simulink model "Sim_Uncertain_Delay_iqctest1"  (Simulink 7.3)
settings: Solver=ode45  StartTime=0.0  StopTime=100.0  RelTol=1e-3
settings Model: Creator=MD710  LastModifiedBy=MD710
settings DebuggingCC: SaveWithParameterizedLinksMsg=none  SolverPrmCheckMsg=none  MultiTaskDSMMsg=warning  MultiTaskCondExecSysMsg=none  FcnCallInpInsideContextMsg=Enable All  StrictBusMsg=None
settings HardwareCC: TargetHWDeviceType=32-bit Generic
settings RTWCC: IncludeERTFirstTime=on
settings GRTTargetCC: TargetFcnLib=ansi_tfl_tmw.mat

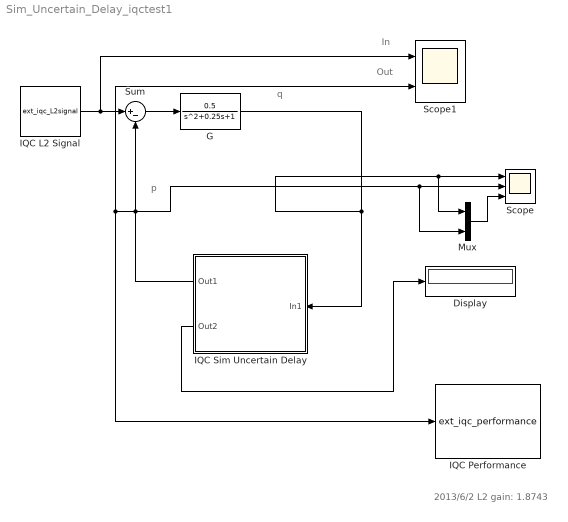
== system Sim_Uncertain_Delay_iqctest1 ==
  note: q
  note: p
  note: 2013/6/2 L2 gain: 1.8743
  note: In
  note: Out
  Display : Display
  G : TransferFcn  Numerator=[0.5]  Denominator=[1 0.25 1]
  IQC L2 Signal : M-S-Function  FunctionName=ext_iqc_L2signal  Parameters=sig_size,sam_time,sig_type,tru_time,sig_amp,sig_fre,user_cus  mask(IQC L2 signal(ver:0.1)){sig_size=1, sam_time=0, sig_type=Step, tru_time=3, sig_amp=1, sig_fre=1, user_cus='2*exp(3*t)'}
      mask prompts: sig_size "Signal Dimension:(Default: 1)"; sam_time "Sample Time:(Default: 0)"; sig_type "Signal Type:"; tru_time "Truncation Time:"; sig_amp "Maximum Amplitude:"; sig_fre "Frequency:"; user_cus "Custom:"
      mask help:
      | Important:
      | In IQC procedure step (as commond iqc_gain_tbx, the task is get
      | L2 gain value), regardless of the user to choose which option (ex sine...),
      | here regarded as generalized L2 signal.
      mask StyleString: edit,edit,popup(Step|Square wave|Sine wave|Custom|Random|External),edit,edit,edit,edit
      mask CallbackString: ||iqc_block_cho(gcb,'L2signal_type')||||
      mask TabNameString: Main,Main,Simulation,Simulation,Simulation,Simulation,Simulation
      mask Display: plot(0:0.1:10,[sin(0:0.1:6.2) zeros(1,38)])
  IQC Performance : M-S-Function  FunctionName=ext_iqc_performance  Parameters=imp_met,save_lin_com,isiqcbode,fre_ran,uselmitool,lmi_par  mask(IQC Performance(ver:0.1)){imp_met=Calculation and Simulation, save_lin_com=off, isiqcbode=off, fre_ran='', uselmitool=lmilab, lmi_par=''}
      mask prompts: imp_met "Implementation Methods"; save_lin_com "Save the Linear File and Command File"; isiqcbode "Display IQC Bode Figure"; fre_ran "Frequency Range:(Default: empty)"; uselmitool "LMI Tool:"; lmi_par "Parameter:(if empty use define)"
      mask help:
      | Important:
      | In IQC toolbox calculate step (as commond iqc_gain_tbx, the task is get
      | L2 gain value), regardless of the user to connect any signal input(Even if
      | not a signal), here regarded as generalized L2 signal.
      |
      | Example 1: setlmioptions('',[0 200 0 0 777])
      | the block parameter is
      | LMI Tool: lmilab
      | Parameter:
      |        [0 200 0 0 777]
      |
      | Example 2: setlmioptions('yalmip','solver','sdpt3','verbose',1)
      | the block parameter is
      | LMI Tool: yalmip
      | Parameter:
      |        {'solver',sdpt3','verbose',1}
      mask Help:
      | <a href="matlab:doc abst_init_iqc;">abst_init_iqc</a>
      | <a href="matlab:doc setlmioptions;">setlmioptions</a>
      | <a href="matlab:doc iqc_gain_tbx;">iqc_gain_tbx</a>
      mask StyleString: popup(Calculation and Simulation|Only Calculation|Only Simulation),checkbox,checkbox,edit,popup(lmilab|yalmip),edit
      mask CallbackString: iqc_block_cho(gcb,'performance_imp')||iqc_block_cho(gcb,'performance_bodefre')|||
      mask TabNameString: Main,Main,Main,Main,LMI,LMI
      mask Display: fprintf('In -> Out \n performance \n L2 gain:\n%4.4f',1.8743);
  IQC Sim Uncertain Delay : Subsystem  mask(IQC Sim Uncertain Delay(ver:0.1)){sou_del=Custom, max_del=0.5, num_ran=1, cus=[0.5], iqc1=on, iqc1_pole=[1 2], iqc1_out='', iqc2=off, iqc2_pole=[], iqc2_out='', iqc3=off, lis_rel='', delay_time=0}
      mask prompts: sou_del "Source of the delay:(Default: Random)"; max_del "Maximum Delay:"; num_ran "The Number of Random:(1 or input_dim)"; cus "Custom:"; iqc1 "iqc_delay(Input,Maximum Delay,Pole)"; iqc1_pole "Pole:(Default: [])"; iqc1_out "Output Variable:(Default: empty)"; iqc2 "iqc_delay1(Input,Maximum Delay,Pole)"; iqc2_pole "Pole:(Default: [])"; iqc2_out "Output Variable:(Default: empty)"; iqc3 "Custom IQC"; lis_rel "List of IQC Relationships:"; delay_time "Mask Parameter 13:"
      mask init:
      | switch sou_del
      |     case 1
      |         delay_time=max_del*rand(1,num_ran);
      |     case 2
      |         delay_time=reshape(cus,1,length(cus));
      | end
      | % fprintf('The Random Delay Time: %4.3f \n',delay_time);
      mask Help:
      | <a href="matlab:doc iqc_delay;">iqc_delay</a>
      | <a href="matlab:doc iqc_delay1;">iqc_delay1</a>
      mask StyleString: popup(Random|Custom),edit,edit,edit,checkbox,edit,edit,checkbox,edit,edit,checkbox,edit,edit
      mask CallbackString: iqc_block_cho(gcb,'sim_uncertaindelay_sou')||||iqc_block_cho(gcb,'sim_uncertaindelay_iqc1')|||iqc_block_cho(gcb,'sim_uncertaindelay_iqc2')|||iqc_block_cho(gcb,'sim_uncertaindelay_iqc3')||
      mask TabNameString: Simulink Parameters,Simulink Parameters,Simulink Parameters,Simulink Parameters,Procedure Parameters,Procedure Parameters,Procedure Parameters,Procedure Parameters,Procedure Parameters,Procedure Parameters,Procedure Parameters,Procedure Parameters,Simulink Parameters
      mask Display: disp('\fontsize{14}exp(-T*s)', 'texmode','on');port_label('input',1,'in');port_label('output',1,'out');port_label('output',2,'T');
  Mux : Mux  Inputs=2
  Scope : Scope  NumInputPorts=3
      settings: YMin=-5~-5~-5  YMax=5~5~5
  Scope1 : Scope  NumInputPorts=2
      settings: YMin=-5~-5  YMax=5~5  SaveName=ScopeData2
  Sum : Sum  Inputs=|+-
  wires:
  IQC L2 Signal/1 -> Scope1/1, Sum/1
  Sum/1 -> G/1
  G/1 -> IQC Sim Uncertain Delay/1(In1), Mux/1, Scope/1
  IQC Sim Uncertain Delay/1(Out1) -> Mux/2, Scope/2, Sum/2, IQC Performance/1, Scope1/2
  IQC Sim Uncertain Delay/2(Out2) -> Display/1
  Mux/1 -> Scope/3

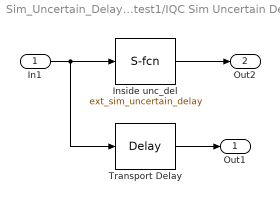
== system Sim_Uncertain_Delay_iqctest1/IQC Sim Uncertain Delay ==
  In1 : Inport
  Inside unc_del : M-S-Function  FunctionName=ext_sim_uncertain_delay  Parameters=sou_del,max_del,num_ran,cus,iqc1,iqc1_pole,iqc1_out,iqc2,iqc2_pole,iqc2_out,iqc3,lis_rel,delay_time
  Transport Delay : TransportDelay  DelayTime=delay_time
  Out1 : Outport
  Out2 : Outport  Port=2
  wires:
  Inside unc_del/1 -> Out2/1
  Transport Delay/1 -> Out1/1
  In1/1 -> Transport Delay/1, Inside unc_del/1
